simulink model "Simple_2Quad_payload_04"  (R2018b)
settings: Solver=VariableStepAuto  StartTime=0.0  StopTime=60  RelTol=1e-3
InitFcn:
  | Simple_2Quad_payload_04_const
values from neighbouring files (symbols this model uses):
  d = 1    [Simple_2Quad_payload_01_const.m]    (also in Simple_2Quad_payload_02_const.m; Simple_2Quad_payload_03_const.m; Simple_2Quad_payload_04_const.m)
  g = 9.81    [Colab_4Quad_model_01_const.m]    (also in Colab_4Quad_model_02_const.m; Simple_2Quad_payload_01_const.m; Simple_2Quad_payload_02_const.m; Simple_2Quad_payload_03_const.m)
  I = 1    [Simple_2Quad_payload_01_const.m]    (also in Simple_2Quad_payload_02_const.m; Simple_2Quad_payload_03_const.m; Simple_2Quad_payload_04_const.m)
  l = 3.1819    [Colab_4Quad_model_01_const.m]    (also in Colab_4Quad_model_02_const.m = 3; Simple_2Quad_payload_04_const.m = 1; Simple_4Quad_payload_01_const.m = 1; Simple_4Quad_payload_02_const.m = 2)
  m = 1.5    [Colab_4Quad_model_01_const.m]    (also in Colab_4Quad_model_02_const.m; Simple_2Quad_payload_04_const.m = 1; Simple_4Quad_payload_01_const.m = 1; Simple_4Quad_payload_02_const.m = 1)
  M = 1.0    (= 1)    [Colab_4Quad_model_01_const.m]    (also in Colab_4Quad_model_02_const.m; Simple_2Quad_payload_01_const.m; Simple_2Quad_payload_02_const.m; Simple_2Quad_payload_03_const.m)
  Md = 1*[1;1;1]    [Simple_2Quad_payload_04_const.m]    (also in Simple_4Quad_payload_01_const.m = 1*[1;1;1;1;1;1]; Simple_4Quad_payload_02_const.m = 1*[1;1;1;1;1;1]; Simple_4Quad_payload_03_const.m = 1*[1;1;1;1;1;1]; Simple_4Quad_payload_04_const.m = 1*[1;1;1;1;1;1])
libraries: simulink x4
settings Model: Creator=ali  LastModifiedBy=ali

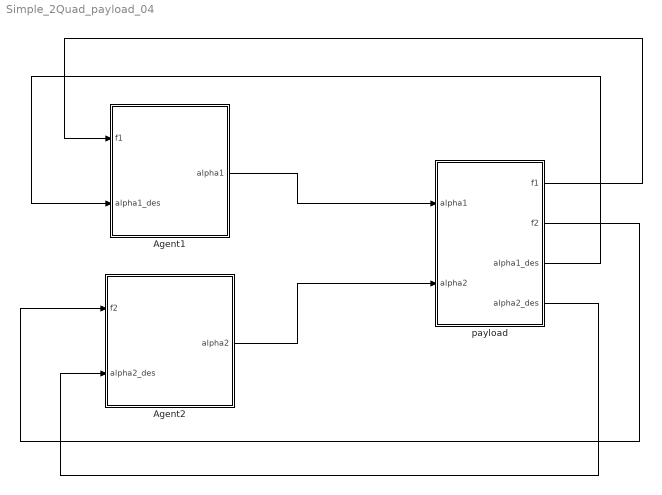
== system Simple_2Quad_payload_04 ==
  "Agent1 " : Subsystem
  Agent2 : Subsystem
  payload : Subsystem
  wires:
  "Agent1 "/1(alpha1) -> payload/1(alpha1)
  payload/1(f1) -> "Agent1 "/1(f1)
  payload/4(alpha2_des) -> Agent2/2(alpha2_des)
  payload/2(f2) -> Agent2/1(f2)
  payload/3(alpha1_des) -> "Agent1 "/2(alpha1_des)
  Agent2/1(alpha2) -> payload/2(alpha2)

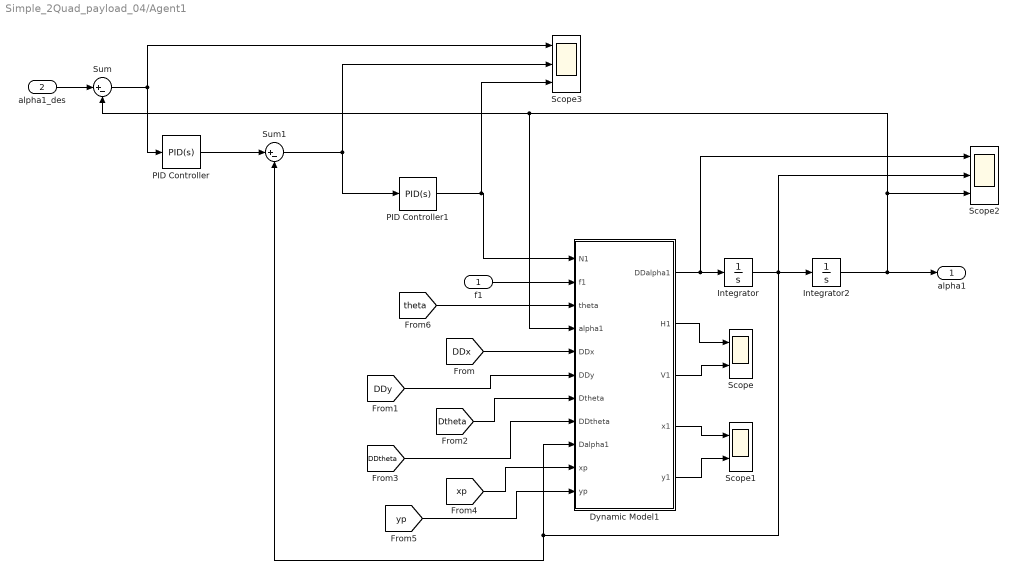
== system Simple_2Quad_payload_04/Agent1  ==
  f1 : Inport
  alpha1_des : Inport  Port=2
  Dynamic Model1 : MATLAB Function  TreatAsAtomicUnit=on
  Integrator : Integrator
  Integrator2 : Integrator  InitialCondition=pi/2
  PID Controller : simulink/Continuous/PID Controller  Controller=PID  Form=Parallel  TimeDomain=Continuous-time  SampleTime=-1  IntegratorMethod=Forward Euler  FilterMethod=Forward Euler  ControllerParametersSource=internal  P=10  I=1  D=0  UseFilter=on  N=100  TunerSelectOption=Transfer Function Based (PID Tuner App)  InitialConditionSource=internal  InitialConditionForIntegrator=0  InitialConditionForFilter=0  DifferentiatorICPrevScaledInput=0  ExternalReset=none  TrackingMode=off  Kt=1  LimitOutput=off  UpperSaturationLimit=inf  LowerSaturationLimit=-inf  LinearizeAsGain=on  AntiWindupMode=none  Kb=1  POutMin=[]  POutMax=[]  IOutMin=[]  IOutMax=[]  DOutMin=[]  DOutMax=[]  NOutMin=[]  NOutMax=[]  SumOutMin=[]  SumOutMax=[]  SaturationOutMin=[]  SaturationOutMax=[]  PParamMin=[]  PParamMax=[]  IParamMin=[]  IParamMax=[]  DParamMin=[]  DParamMax=[]  NParamMin=[]  NParamMax=[]  KbParamMin=[]  KbParamMax=[]  KtParamMin=[]  KtParamMax=[]  KbOutMin=[]  KbOutMax=[]  KtOutMin=[]  KtOutMax=[]  IntegratorOutMin=[]  IntegratorOutMax=[]  FilterOutMin=[]  FilterOutMax=[]  SumI1OutMin=[]  SumI1OutMax=[]  SumI2OutMin=[]  SumI2OutMax=[]  SumI3OutMin=[]  SumI3OutMax=[]  SumI4OutMin=[]  SumI4OutMax=[]  SumDOutMin=[]  SumDOutMax=[]  DifferentiatorOutMin=[]  DifferentiatorOutMax=[]  FilterDiffOutCoefMin=[]  FilterDiffOutCoefMax=[]  ReciprocalOutMin=[]  ReciprocalOutMax=[]  SumDenOutMin=[]  SumDenOutMax=[]  SumNumOutMin=[]  SumNumOutMax=[]  DivideOutMin=[]  DivideOutMax=[]  IntegratorContinuousStateAttributes=''  IntegratorStateMustResolveToSignalObject=off  IntegratorRTWStateStorageClass=Auto  FilterContinuousStateAttributes=''  FilterStateMustResolveToSignalObject=off  FilterRTWStateStorageClass=Auto  ParallelPVariant=InternalParameters  IdealPVariant=Disabled  IVariant=InternalParameters  DVariant=InternalParameters  IntegratorVariant=Continuous  SatVariant=Disabled  AWVariant=Passthrough  PCopyVariant=Disabled  TRVariant=Disabled  FdbkBlocksVariant=Forward  IdealPFdbkVariant=Disabled  SatFdbkVariant=Disabled  DerivativeFilterVariant=ContFilter  NVariant=InternalParameters  NCopyVariant=Disabled  FilterICVariant=InternalICsFilter  IntegratorICVariant=InternalICs  ExternalResetVariant=Disabled  TRSumVariant=Passthrough  SumFdbkVariant=Disabled  SumVariant=Sum_PID
  PID Controller1 : simulink/Continuous/PID Controller  Controller=PID  Form=Parallel  TimeDomain=Continuous-time  SampleTime=-1  IntegratorMethod=Forward Euler  FilterMethod=Forward Euler  ControllerParametersSource=internal  P=100  I=0  D=0  UseFilter=on  N=100  TunerSelectOption=Transfer Function Based (PID Tuner App)  InitialConditionSource=internal  InitialConditionForIntegrator=0  InitialConditionForFilter=0  DifferentiatorICPrevScaledInput=0  ExternalReset=none  TrackingMode=off  Kt=1  LimitOutput=off  UpperSaturationLimit=inf  LowerSaturationLimit=-inf  LinearizeAsGain=on  AntiWindupMode=none  Kb=1  POutMin=[]  POutMax=[]  IOutMin=[]  IOutMax=[]  DOutMin=[]  DOutMax=[]  NOutMin=[]  NOutMax=[]  SumOutMin=[]  SumOutMax=[]  SaturationOutMin=[]  SaturationOutMax=[]  PParamMin=[]  PParamMax=[]  IParamMin=[]  IParamMax=[]  DParamMin=[]  DParamMax=[]  NParamMin=[]  NParamMax=[]  KbParamMin=[]  KbParamMax=[]  KtParamMin=[]  KtParamMax=[]  KbOutMin=[]  KbOutMax=[]  KtOutMin=[]  KtOutMax=[]  IntegratorOutMin=[]  IntegratorOutMax=[]  FilterOutMin=[]  FilterOutMax=[]  SumI1OutMin=[]  SumI1OutMax=[]  SumI2OutMin=[]  SumI2OutMax=[]  SumI3OutMin=[]  SumI3OutMax=[]  SumI4OutMin=[]  SumI4OutMax=[]  SumDOutMin=[]  SumDOutMax=[]  DifferentiatorOutMin=[]  DifferentiatorOutMax=[]  FilterDiffOutCoefMin=[]  FilterDiffOutCoefMax=[]  ReciprocalOutMin=[]  ReciprocalOutMax=[]  SumDenOutMin=[]  SumDenOutMax=[]  SumNumOutMin=[]  SumNumOutMax=[]  DivideOutMin=[]  DivideOutMax=[]  IntegratorContinuousStateAttributes=''  IntegratorStateMustResolveToSignalObject=off  IntegratorRTWStateStorageClass=Auto  FilterContinuousStateAttributes=''  FilterStateMustResolveToSignalObject=off  FilterRTWStateStorageClass=Auto  ParallelPVariant=InternalParameters  IdealPVariant=Disabled  IVariant=InternalParameters  DVariant=InternalParameters  IntegratorVariant=Continuous  SatVariant=Disabled  AWVariant=Passthrough  PCopyVariant=Disabled  TRVariant=Disabled  FdbkBlocksVariant=Forward  IdealPFdbkVariant=Disabled  SatFdbkVariant=Disabled  DerivativeFilterVariant=ContFilter  NVariant=InternalParameters  NCopyVariant=Disabled  FilterICVariant=InternalICsFilter  IntegratorICVariant=InternalICs  ExternalResetVariant=Disabled  TRSumVariant=Passthrough  SumFdbkVariant=Disabled  SumVariant=Sum_PID
  Scope : Scope  NumInputPorts=2
  Scope1 : Scope  NumInputPorts=2
  Scope2 : Scope  NumInputPorts=3
  Scope3 : Scope  NumInputPorts=3
  Sum : Sum  Inputs=|+-
  Sum1 : Sum  Inputs=|+-
  alpha1 : Outport
  wires:
  Dynamic Model1/1(DDalpha1) -> Scope2/1, Integrator/1
  Integrator/1 -> Scope2/2, Sum1/2, Dynamic Model1/9(Dalpha1), Integrator2/1
  [theta] -> Dynamic Model1/3(theta)
  f1/1 -> Dynamic Model1/2(f1)
  Sum/1 -> Scope3/1, PID Controller/1
  alpha1_des/1 -> Sum/1
  Integrator2/1 -> alpha1/1, Scope2/3, Dynamic Model1/4(alpha1), Sum/2
  Dynamic Model1/2(H1) -> Scope/1
  Dynamic Model1/3(V1) -> Scope/2
  Dynamic Model1/4(x1) -> Scope1/1
  Dynamic Model1/5(y1) -> Scope1/2
  [DDx] -> Dynamic Model1/5(DDx)
  [DDy] -> Dynamic Model1/6(DDy)
  [Dtheta] -> Dynamic Model1/7(Dtheta)
  [DDtheta] -> Dynamic Model1/8(DDtheta)
  [xp] -> Dynamic Model1/10(xp)
  [yp] -> Dynamic Model1/11(yp)
  PID Controller1/1 -> Scope3/3, Dynamic Model1/1(N1)
  PID Controller/1 -> Sum1/1
  Sum1/1 -> Scope3/2, PID Controller1/1

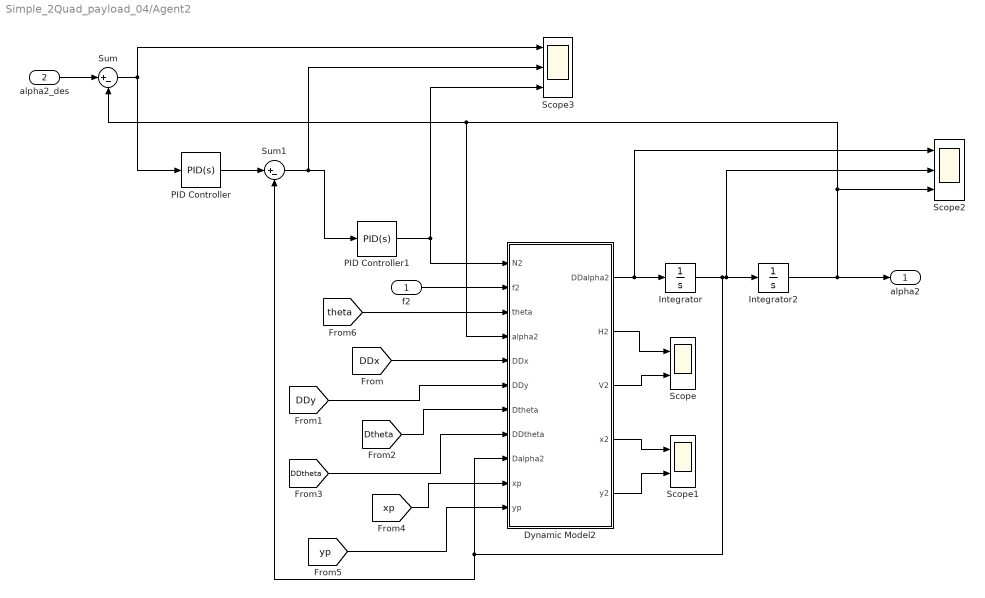
== system Simple_2Quad_payload_04/Agent2 ==
  f2 : Inport
  alpha2_des : Inport  Port=2
  Dynamic Model2 : MATLAB Function  TreatAsAtomicUnit=on
  Integrator : Integrator
  Integrator2 : Integrator  InitialCondition=pi/2
  PID Controller : simulink/Continuous/PID Controller  Controller=PID  Form=Parallel  TimeDomain=Continuous-time  SampleTime=-1  IntegratorMethod=Forward Euler  FilterMethod=Forward Euler  ControllerParametersSource=internal  P=10  I=1  D=0  UseFilter=on  N=100  TunerSelectOption=Transfer Function Based (PID Tuner App)  InitialConditionSource=internal  InitialConditionForIntegrator=0  InitialConditionForFilter=0  DifferentiatorICPrevScaledInput=0  ExternalReset=none  TrackingMode=off  Kt=1  LimitOutput=off  UpperSaturationLimit=inf  LowerSaturationLimit=-inf  LinearizeAsGain=on  AntiWindupMode=none  Kb=1  POutMin=[]  POutMax=[]  IOutMin=[]  IOutMax=[]  DOutMin=[]  DOutMax=[]  NOutMin=[]  NOutMax=[]  SumOutMin=[]  SumOutMax=[]  SaturationOutMin=[]  SaturationOutMax=[]  PParamMin=[]  PParamMax=[]  IParamMin=[]  IParamMax=[]  DParamMin=[]  DParamMax=[]  NParamMin=[]  NParamMax=[]  KbParamMin=[]  KbParamMax=[]  KtParamMin=[]  KtParamMax=[]  KbOutMin=[]  KbOutMax=[]  KtOutMin=[]  KtOutMax=[]  IntegratorOutMin=[]  IntegratorOutMax=[]  FilterOutMin=[]  FilterOutMax=[]  SumI1OutMin=[]  SumI1OutMax=[]  SumI2OutMin=[]  SumI2OutMax=[]  SumI3OutMin=[]  SumI3OutMax=[]  SumI4OutMin=[]  SumI4OutMax=[]  SumDOutMin=[]  SumDOutMax=[]  DifferentiatorOutMin=[]  DifferentiatorOutMax=[]  FilterDiffOutCoefMin=[]  FilterDiffOutCoefMax=[]  ReciprocalOutMin=[]  ReciprocalOutMax=[]  SumDenOutMin=[]  SumDenOutMax=[]  SumNumOutMin=[]  SumNumOutMax=[]  DivideOutMin=[]  DivideOutMax=[]  IntegratorContinuousStateAttributes=''  IntegratorStateMustResolveToSignalObject=off  IntegratorRTWStateStorageClass=Auto  FilterContinuousStateAttributes=''  FilterStateMustResolveToSignalObject=off  FilterRTWStateStorageClass=Auto  ParallelPVariant=InternalParameters  IdealPVariant=Disabled  IVariant=InternalParameters  DVariant=InternalParameters  IntegratorVariant=Continuous  SatVariant=Disabled  AWVariant=Passthrough  PCopyVariant=Disabled  TRVariant=Disabled  FdbkBlocksVariant=Forward  IdealPFdbkVariant=Disabled  SatFdbkVariant=Disabled  DerivativeFilterVariant=ContFilter  NVariant=InternalParameters  NCopyVariant=Disabled  FilterICVariant=InternalICsFilter  IntegratorICVariant=InternalICs  ExternalResetVariant=Disabled  TRSumVariant=Passthrough  SumFdbkVariant=Disabled  SumVariant=Sum_PID
  PID Controller1 : simulink/Continuous/PID Controller  Controller=PID  Form=Parallel  TimeDomain=Continuous-time  SampleTime=-1  IntegratorMethod=Forward Euler  FilterMethod=Forward Euler  ControllerParametersSource=internal  P=100  I=0  D=0  UseFilter=on  N=100  TunerSelectOption=Transfer Function Based (PID Tuner App)  InitialConditionSource=internal  InitialConditionForIntegrator=0  InitialConditionForFilter=0  DifferentiatorICPrevScaledInput=0  ExternalReset=none  TrackingMode=off  Kt=1  LimitOutput=off  UpperSaturationLimit=inf  LowerSaturationLimit=-inf  LinearizeAsGain=on  AntiWindupMode=none  Kb=1  POutMin=[]  POutMax=[]  IOutMin=[]  IOutMax=[]  DOutMin=[]  DOutMax=[]  NOutMin=[]  NOutMax=[]  SumOutMin=[]  SumOutMax=[]  SaturationOutMin=[]  SaturationOutMax=[]  PParamMin=[]  PParamMax=[]  IParamMin=[]  IParamMax=[]  DParamMin=[]  DParamMax=[]  NParamMin=[]  NParamMax=[]  KbParamMin=[]  KbParamMax=[]  KtParamMin=[]  KtParamMax=[]  KbOutMin=[]  KbOutMax=[]  KtOutMin=[]  KtOutMax=[]  IntegratorOutMin=[]  IntegratorOutMax=[]  FilterOutMin=[]  FilterOutMax=[]  SumI1OutMin=[]  SumI1OutMax=[]  SumI2OutMin=[]  SumI2OutMax=[]  SumI3OutMin=[]  SumI3OutMax=[]  SumI4OutMin=[]  SumI4OutMax=[]  SumDOutMin=[]  SumDOutMax=[]  DifferentiatorOutMin=[]  DifferentiatorOutMax=[]  FilterDiffOutCoefMin=[]  FilterDiffOutCoefMax=[]  ReciprocalOutMin=[]  ReciprocalOutMax=[]  SumDenOutMin=[]  SumDenOutMax=[]  SumNumOutMin=[]  SumNumOutMax=[]  DivideOutMin=[]  DivideOutMax=[]  IntegratorContinuousStateAttributes=''  IntegratorStateMustResolveToSignalObject=off  IntegratorRTWStateStorageClass=Auto  FilterContinuousStateAttributes=''  FilterStateMustResolveToSignalObject=off  FilterRTWStateStorageClass=Auto  ParallelPVariant=InternalParameters  IdealPVariant=Disabled  IVariant=InternalParameters  DVariant=InternalParameters  IntegratorVariant=Continuous  SatVariant=Disabled  AWVariant=Passthrough  PCopyVariant=Disabled  TRVariant=Disabled  FdbkBlocksVariant=Forward  IdealPFdbkVariant=Disabled  SatFdbkVariant=Disabled  DerivativeFilterVariant=ContFilter  NVariant=InternalParameters  NCopyVariant=Disabled  FilterICVariant=InternalICsFilter  IntegratorICVariant=InternalICs  ExternalResetVariant=Disabled  TRSumVariant=Passthrough  SumFdbkVariant=Disabled  SumVariant=Sum_PID
  Scope : Scope  NumInputPorts=2
  Scope1 : Scope  NumInputPorts=2
  Scope2 : Scope  NumInputPorts=3
  Scope3 : Scope  NumInputPorts=3
  Sum : Sum  Inputs=|+-
  Sum1 : Sum  Inputs=|+-
  alpha2 : Outport
  wires:
  Dynamic Model2/5(y2) -> Scope1/2
  Dynamic Model2/4(x2) -> Scope1/1
  Dynamic Model2/3(V2) -> Scope/2
  Dynamic Model2/2(H2) -> Scope/1
  alpha2_des/1 -> Sum/1
  PID Controller1/1 -> Dynamic Model2/1(N2), Scope3/3
  f2/1 -> Dynamic Model2/2(f2)
  [theta] -> Dynamic Model2/3(theta)
  Dynamic Model2/1(DDalpha2) -> Scope2/1, Integrator/1
  [yp] -> Dynamic Model2/11(yp)
  [DDy] -> Dynamic Model2/6(DDy)
  [Dtheta] -> Dynamic Model2/7(Dtheta)
  [DDtheta] -> Dynamic Model2/8(DDtheta)
  [DDx] -> Dynamic Model2/5(DDx)
  [xp] -> Dynamic Model2/10(xp)
  Sum1/1 -> Scope3/2, PID Controller1/1
  Integrator/1 -> Scope2/2, Integrator2/1, Sum1/2, Dynamic Model2/9(Dalpha2)
  PID Controller/1 -> Sum1/1
  Integrator2/1 -> Scope2/3, Sum/2, Dynamic Model2/4(alpha2), alpha2/1
  Sum/1 -> Scope3/1, PID Controller/1

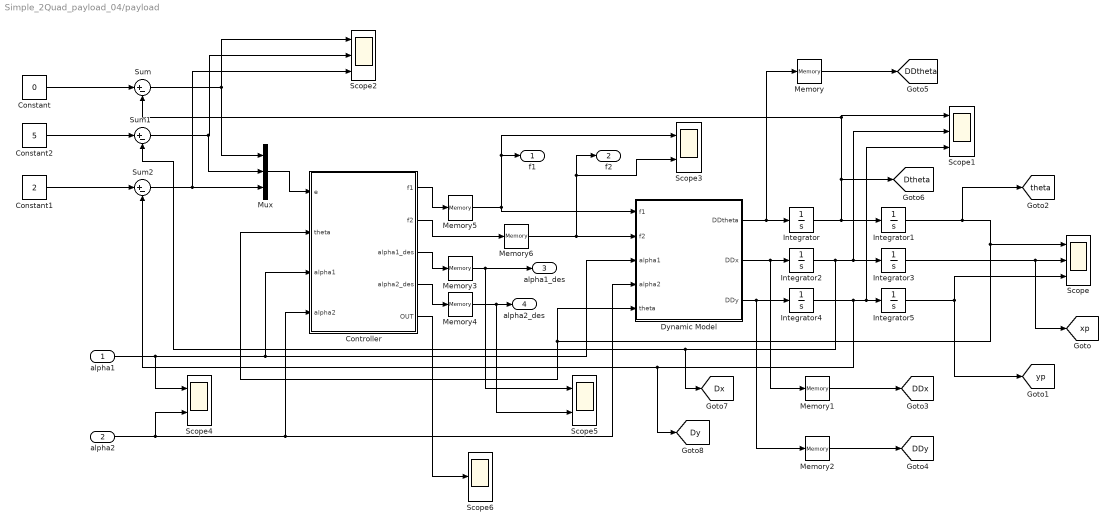
== system Simple_2Quad_payload_04/payload ==
  alpha1 : Inport
  alpha2 : Inport  Port=2
  Constant : Constant  Value=0
  Constant1 : Constant  Value=2
  Constant2 : Constant  Value=5
  Controller : MATLAB Function  TreatAsAtomicUnit=on
  Dynamic Model : MATLAB Function  TreatAsAtomicUnit=on
  Integrator{,1..4} (5 alike) : Integrator
  Integrator5 : Integrator  InitialCondition=10
  Memory{,1..6} (7 alike) : Memory
  Mux : Mux  Inputs=3
  Scope : Scope  NumInputPorts=3
  Scope1 : Scope  NumInputPorts=3
  Scope2 : Scope  NumInputPorts=3
  Scope3 : Scope  NumInputPorts=2
  Scope4 : Scope  NumInputPorts=2
  Scope5 : Scope  NumInputPorts=2
  Scope6 : Scope
  Sum : Sum  Inputs=|+-
  Sum1 : Sum  Inputs=|+-
  Sum2 : Sum  Inputs=|+-
  f1 : Outport
  f2 : Outport  Port=2
  alpha1_des : Outport  Port=3
  alpha2_des : Outport  Port=4
  tag scope: DDtheta=global, DDx=global, DDy=global, Dtheta=global, Dx=global, Dy=global, theta=global, xp=global, yp=global
  wires:
  Controller/3(alpha1_des) -> Memory3/1
  Controller/4(alpha2_des) -> Memory4/1
  Dynamic Model/1(DDtheta) -> Memory/1, Integrator/1
  Integrator/1 -> [Dtheta], Scope1/1, Sum/2, Integrator1/1
  Integrator1/1 -> [theta], Scope/1, Controller/2(theta), Dynamic Model/5(theta)
  Integrator2/1 -> [Dx], Sum1/2, Scope1/2, Integrator3/1
  Dynamic Model/2(DDx) -> Integrator2/1, Memory1/1
  Integrator4/1 -> Scope1/3, Integrator5/1, [Dy], Sum2/2
  Dynamic Model/3(DDy) -> Integrator4/1, Memory2/1
  alpha1/1 -> Dynamic Model/3(alpha1), Controller/3(alpha1), Scope4/1
  alpha2/1 -> Controller/4(alpha2), Dynamic Model/4(alpha2), Scope4/2
  Integrator3/1 -> [xp], Scope/2
  Integrator5/1 -> Scope/3, [yp]
  Sum2/1 -> Mux/3, Scope2/3
  Sum/1 -> Mux/1, Scope2/1
  Constant/1 -> Sum/1
  Constant2/1 -> Sum1/1
  Constant1/1 -> Sum2/1
  Sum1/1 -> Mux/2, Scope2/2
  Memory/1 -> [DDtheta]
  Memory1/1 -> [DDx]
  Memory2/1 -> [DDy]
  Memory3/1 -> Scope5/1, alpha1_des/1
  Memory4/1 -> Scope5/2, alpha2_des/1
  Controller/1(f1) -> Memory5/1
  Controller/2(f2) -> Memory6/1
  Memory5/1 -> Dynamic Model/1(f1), Scope3/1, f1/1
  Memory6/1 -> Scope3/2, f2/1, Dynamic Model/2(f2)
  Controller/5(OUT) -> Scope6/1
  Mux/1 -> Controller/1(e)

== matlab function Simple_2Quad_payload_04/payload/Controller ==
  data: e input; f1 output; theta input; alpha1 input; alpha2 input; f2 output; alpha1_des output; alpha2_des output; Md parameter; g parameter; M parameter; d parameter; I parameter; OUT output
function [f1,f2,alpha1_des,alpha2_des,OUT] = fcn(e,theta,alpha1,alpha2, Md, g, M, d, I)

A = [(d/I) 0 0;
    0 (1/M)*cos(theta) (-1/M)*sin(theta);
    0 (1/M)*sin(theta) (1/M)*cos(theta)];

B = [sin(alpha1) -sin(alpha2);
    cos(alpha1) cos(alpha2);
    sin(alpha1) sin(alpha2)];

D = [0;0;-g];

%SGN = diag(sign(e));
SGN = zeros(3);
for i=1:3
    SGN(i,i) = e(i)/(abs(e(i))+0.5);
end

Z = SGN*Md;
U = Z - D;
F = ((B'*(A'*A)*B)^(-1))*(B'*A')*U;

f1 = F(1);
f2 = F(2);

alpha1_des = atan((U(3)/(U(2)+0.01)));
alpha2_des = atan((U(3)/(U(2)+0.01)));

OUT = U;

end

== matlab function Simple_2Quad_payload_04/payload/Dynamic Model ==
  data: f1 input; DDtheta output; f2 input; alpha1 input; alpha2 input; theta input; DDx output; DDy output; d parameter; M parameter; I parameter; g parameter
function [DDtheta,DDx,DDy] = fcn(f1,f2,alpha1,alpha2,theta,d, M, I, g)

DDtheta = (d/I) * ( f1*sin(alpha1) - f2*sin(alpha2) );
DDx = (1/M) * ( f1*cos(alpha1+theta) + f2*cos(alpha2+theta) );
DDy = (1/M) * ( f1*sin(alpha1+theta) + f2*sin(alpha2+theta) - (M*g) );

end

== matlab function Simple_2Quad_payload_04/Agent2/Dynamic Model2 ==
  data: DDalpha2 output; N2 input; f2 input; theta input; alpha2 input; m parameter; g parameter; DDx input; DDy input; Dtheta input; DDtheta input; Dalpha2 input; H2 output; V2 output; l parameter; d parameter; xp input; yp input; x2 output; y2 output
function [DDalpha2,H2,V2,x2,y2]  = fcn(N2,f2,theta,alpha2,m, g,DDx,DDy,Dtheta,DDtheta,Dalpha2, l, d,xp,yp)

DDalpha2 = (1/m/l) * ( N2 - (m*g*cos(alpha2)) + (DDx*sin(theta+alpha2)) - (DDy*cos(theta+alpha2)) - ((Dtheta^2)*d*sin(alpha2)) - (DDtheta*d*cos(alpha2)) );
T2 = f2 + (m*g*sin(alpha2)) + (m * ( (DDx*cos(theta+alpha2)) + (DDy*sin(theta+alpha2)) - ((Dtheta)^2)*d*cos(alpha2) + (DDtheta*d*sin(alpha2)) - ((Dalpha2^2)*l) ));

H2 = -N2*sin(alpha2+theta) + T2*cos(alpha2+theta);
V2 = N2*cos(alpha2+theta) + T2*sin(alpha2+theta);

x2 = xp - (d*cos(theta)) + (l*cos(alpha2+theta));
y2 = yp - (d*sin(theta)) + (l*sin(alpha2+theta));

end

== matlab function Simple_2Quad_payload_04/Agent1 /Dynamic Model1 ==
  data: DDalpha1 output; N1 input; f1 input; theta input; alpha1 input; m parameter; g parameter; DDx input; DDy input; Dtheta input; DDtheta input; Dalpha1 input; H1 output; V1 output; l parameter; d parameter; xp input; yp input; x1 output; y1 output
function [DDalpha1,H1,V1,x1,y1]  = fcn(N1,f1,theta,alpha1,m, g,DDx,DDy,Dtheta,DDtheta,Dalpha1, l, d,xp,yp)

DDalpha1 = (1/m/l) * ( N1 - (m*g*cos(alpha1)) + (DDx*sin(theta+alpha1)) - (DDy*cos(theta+alpha1)) - ((Dtheta^2)*d*sin(alpha1)) - (DDtheta*d*cos(alpha1)) );
T1 = f1 + (m*g*sin(alpha1)) + (m * ( (DDx*cos(theta+alpha1)) + (DDy*sin(theta+alpha1)) - ((Dtheta)^2)*d*cos(alpha1) + (DDtheta*d*sin(alpha1)) - ((Dalpha1^2)*l) ));

H1 = -N1*sin(alpha1+theta) + T1*cos(alpha1+theta);
V1 = N1*cos(alpha1+theta) + T1*sin(alpha1+theta);

x1 = xp + (d*cos(theta)) + (l*cos(alpha1+theta));
y1 = yp + (d*sin(theta)) + (l*sin(alpha1+theta));

end
